simulink model "Practica6_Simulink"  (R2022b)
settings: Solver=VariableStepAuto  StartTime=0.0  StopTime=0.003  MaxStep=0.0000001  RelTol=1e-3
values from neighbouring files (symbols this model uses):
  C1 = 0.0000001    (= 1e-07)    [Parametros_Practica6.m]    (also in Practica6.m)
  C2 = 0.0000001    (= 1e-07)    [Parametros_Practica6.m]    (also in Practica6.m)
  R1 = 1000    [Parametros_Practica6.m]    (also in Practica6.m)
  R2 = 1000    [Parametros_Practica6.m]    (also in Practica6.m)
  R3 = 10000    [Parametros_Practica6.m]    (also in Practica6.m)
  R4 = 15000    [Parametros_Practica6.m]    (also in Practica6.m)
settings Model: Creator=52466  LastModifiedBy=52466

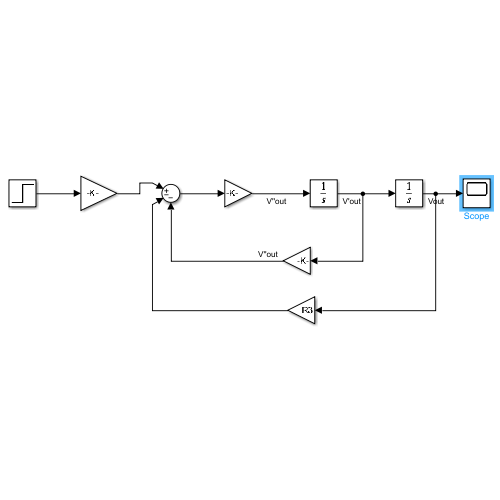
[thumbnail: Simulink's stored preview of the top-level diagram]
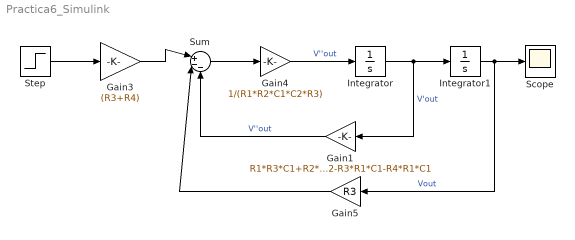
== system Practica6_Simulink ==
  Gain1 : Gain  Gain=R1*R3*C1+R2*R3*C2+R1*R3*C2-R3*R1*C1-R4*R1*C1
  Gain3 : Gain  Gain=(R3+R4)
  Gain4 : Gain  Gain=1/(R1*R2*C1*C2*R3)
  Gain5 : Gain  Gain=R3
  Integrator : Integrator
  Integrator1 : Integrator
  Scope : Scope
  Step : Step  Time=0  SampleTime=0
  Sum : Sum  Inputs=|+--
  wires:
  Step/1 -> Gain3/1
  Gain4/1 -> Integrator/1  "V''out"
  Gain3/1 -> Sum/1
  Integrator/1 -> Gain1/1, Integrator1/1  "V'out"
  Sum/1 -> Gain4/1
  Integrator1/1 -> Gain5/1, Scope/1  "Vout"
  Gain5/1 -> Sum/2
  Gain1/1 -> Sum/3  "V''out"
